simulink model "FuzzyController_SCARA"  (R2023b)
settings: Solver=VariableStepAuto  StartTime=0.0  StopTime=25  RelTol=1e-3
libraries: fuzblock x1
settings Model: Creator=Hamid Reza  LastModifiedBy=Hamid Reza

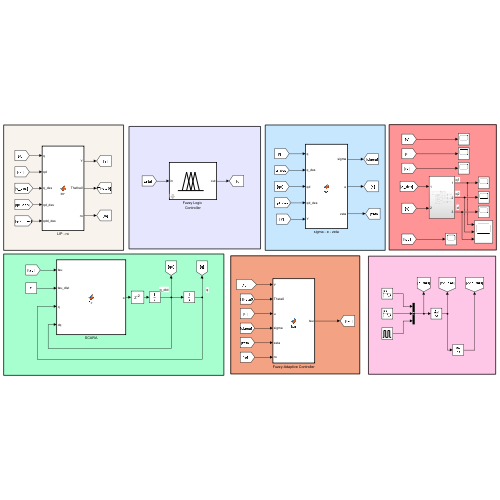
[thumbnail: Simulink's stored preview of the top-level diagram]
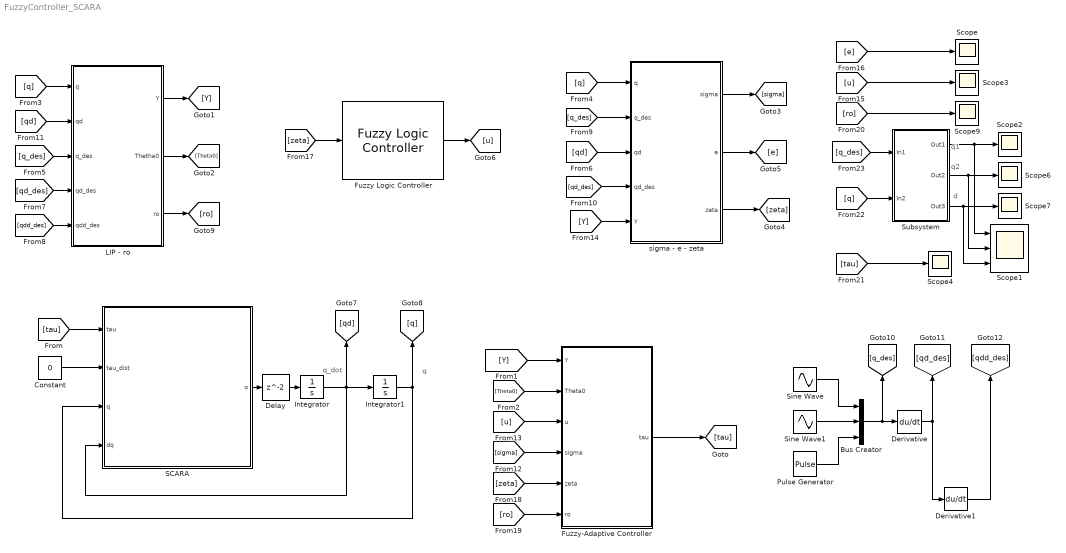
== system FuzzyController_SCARA ==
  note: q_dot
  note: q
  note: q2
  note: d
  note: q1
  Bus Creator : BusCreator  Inputs=3
  Constant : Constant  Value=0
  Delay : Delay
  Derivative : Derivative
  Derivative1 : Derivative
  Fuzzy Logic Controller : fuzblock/Fuzzy Logic  Controller  FIS='scara.fis'  OutputSampleNumber=101  DataType=double  FuzzifiedInputs=off  RuleFiringStrengths=off  RuleOutputs=off  AggregatedOutputs=off  SimulateUsing=Interpreted execution  OutOfRangeInputValueMessage=warning  NoRuleFiredMessage=warning  EmptyOutputFuzzySetMessage=warning
  Fuzzy-Adaptive Controller : MATLAB Function  TreatAsAtomicUnit=on
  Integrator : Integrator  InitialCondition=zeros(3,1)
  Integrator1 : Integrator  InitialCondition=zeros(3,1)
  LIP - ro : MATLAB Function  TreatAsAtomicUnit=on
  Pulse Generator : DiscretePulseGenerator  PulseType=Time based  Period=5  PulseWidth=50
  SCARA : MATLAB Function  TreatAsAtomicUnit=on
  Scope{,2..4,6..7,9} (7 alike) : Scope
  Scope1 : Scope  NumInputPorts=3
  Sine Wave : Sin  Frequency=5  SampleTime=0
  Sine Wave1 : Sin  Frequency=5  Phase=pi/2  SampleTime=0
  Subsystem : Subsystem
  sigma - e - zeta : MATLAB Function  TreatAsAtomicUnit=on
  wires:
  Integrator1/1 -> SCARA/3(q), [q]
  Integrator/1 -> SCARA/4(dq), Integrator1/1, [qd]
  Constant/1 -> SCARA/2(tau_dist)
  [tau] -> SCARA/1(tau)
  Fuzzy-Adaptive Controller/1(tau) -> [tau]
  [Y] -> Fuzzy-Adaptive Controller/1(Y)
  [Theta0] -> Fuzzy-Adaptive Controller/2(Theta0)
  [q] -> sigma - e - zeta/1(q)
  [qd] -> sigma - e - zeta/3(qd)
  [q_des] -> sigma - e - zeta/2(q_des)
  sigma - e - zeta/1(sigma) -> [sigma]
  sigma - e - zeta/2(e) -> [e]
  [qd_des] -> sigma - e - zeta/4(qd_des)
  Sine Wave/1 -> Bus Creator/1
  Sine Wave1/1 -> Bus Creator/2
  Bus Creator/1 -> [q_des], Derivative/1
  Derivative/1 -> Derivative1/1, [qd_des]
  Derivative1/1 -> [qdd_des]
  Pulse Generator/1 -> Bus Creator/3
  [e] -> Scope/1
  [tau] -> Scope4/1
  [q_des] -> Subsystem/1(In1)
  [q] -> Subsystem/2(In2)
  Subsystem/1(Out1) -> Scope2/1, Scope1/1
  Subsystem/2(Out2) -> Scope1/2, Scope6/1
  Subsystem/3(Out3) -> Scope1/3, Scope7/1
  [q] -> LIP - ro/1(q)
  [qdd_des] -> LIP - ro/5(qdd_des)
  [qd_des] -> LIP - ro/4(qd_des)
  [q_des] -> LIP - ro/3(q_des)
  [qd] -> LIP - ro/2(qd)
  LIP - ro/2(Thetha0) -> [Theta0]
  LIP - ro/1(Y) -> [Y]
  [sigma] -> Fuzzy-Adaptive Controller/4(sigma)
  [u] -> Fuzzy-Adaptive Controller/3(u)
  [Y] -> sigma - e - zeta/5(Y)
  sigma - e - zeta/3(zeta) -> [zeta]
  Fuzzy Logic Controller/1 -> [u]
  [zeta] -> Fuzzy Logic Controller/1
  [u] -> Scope3/1
  [zeta] -> Fuzzy-Adaptive Controller/5(zeta)
  SCARA/1(o) -> Delay/1
  Delay/1 -> Integrator/1
  [ro] -> Fuzzy-Adaptive Controller/6(ro)
  LIP - ro/3(ro) -> [ro]
  [ro] -> Scope9/1

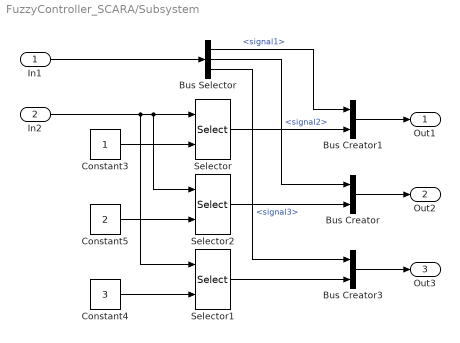
== system FuzzyController_SCARA/Subsystem ==
  In1 : Inport
  In2 : Inport  Port=2
  Bus Creator : BusCreator  Inputs=2
  Bus Creator1 : BusCreator  Inputs=2
  Bus Creator3 : BusCreator  Inputs=2
  Bus Selector : BusSelector  OutputSignals=signal1,signal2,signal3
  Constant3 : Constant
  Constant4 : Constant  Value=3
  Constant5 : Constant  Value=2
  Selector : Selector  InputPortWidth=3  IndexOptions=Index vector (port)  Indices=1  OutputSizes=1
  Selector1 : Selector  InputPortWidth=3  IndexOptions=Index vector (port)  Indices=1  OutputSizes=1
  Selector2 : Selector  InputPortWidth=3  IndexOptions=Index vector (port)  Indices=1  OutputSizes=1
  Out1 : Outport
  Out2 : Outport  Port=2
  Out3 : Outport  Port=3
  wires:
  Bus Selector/3 -> Bus Creator3/1  "<signal3>"
  Bus Selector/2 -> Bus Creator/1  "<signal2>"
  Selector2/1 -> Bus Creator/2
  Constant3/1 -> Selector/2
  Selector/1 -> Bus Creator1/2
  Bus Selector/1 -> Bus Creator1/1  "<signal1>"
  Bus Creator3/1 -> Out3/1
  Selector1/1 -> Bus Creator3/2
  Constant5/1 -> Selector2/2
  Constant4/1 -> Selector1/2
  In2/1 -> Selector1/1, Selector2/1, Selector/1
  Bus Creator/1 -> Out2/1
  Bus Creator1/1 -> Out1/1
  In1/1 -> Bus Selector/1

== matlab function FuzzyController_SCARA/Fuzzy-Adaptive Controller ==
  data: Y input; tau output; Theta0 input; u input; sigma input; zeta input; ro input
function tau = fcn(Y, Theta0, u, sigma, zeta, ro)

tau = (Y*(Theta0 - u)) - K_adaptive(sigma,[0.000001;0.000001;0.000001],zeta,u, ro)*sigma ;



function K = K_adaptive (sigma, epsilon, zeta, u, ro)

    if sigma > epsilon
       K1 = max((abs(zeta).*abs(ro-u))/sigma(1)^2)  ;
       K2 = max((abs(zeta).*abs(ro-u))/sigma(2)^2)  ;
       K3 = max((abs(zeta).*abs(ro-u))/sigma(3)^2)  ;
       K = diag([K1, K2, K3]);
    else
       K = max( (abs(zeta).*abs(ro-u))/epsilon) ;
       K = diag(K);
    end
end

end

== matlab function FuzzyController_SCARA/SCARA ==
  data: tau input; tau_dist input; q input; dq input; o output
function o  = fcn(tau,tau_dist,q,dq)



theta1=q(1);
theta2=q(2);
d=q(3);

dtheta1=dq(1);
dtheta2=dq(2);
dd=dq(3);


a1=0.6;
a2=0.4;
m1=12;
m2=6;
m3=6;
g = 9.81;


% define mass matrix

m11 = (1/3)*m1*a1^2+m2*(a1^2+(1/3)*a2^2+a1*a2*cos(theta2))+m3*(a1^2+a2^2+2*a1*a2*cos(theta2));
m12 = -m2*a2*((1/3)*a2+(1/2)*a1*cos(theta2))-m3*(a2^2+a1*a2*cos(theta2));
m13 = 0;
m21 = m12;
m22 = (1/3)*m2*a2^2+m3*(a2^2);
m23 = 0;
m31 = m13;
m32 = m23;
m33 = m3;

M = [m11,m12,m13;m21,m22,m23;m31,m32,m33];


% define gravity matrix

g = [0; 0; -m3*g];

% define coriolis and centrifugal matrix

c1 = -(m2+2*m3)*a1*a2*sin(theta2)*(dtheta1*dtheta2+((1/2)*dtheta2^2));
c2 = ((1/2)*m2+m3)*a1*a2*sin(theta2)*(dtheta1^2);
c3 = 0;

C = [c1 ; c2 ; c3];


o=pinv(M)*(tau+tau_dist-(C+g));

== matlab function FuzzyController_SCARA/LIP - ro ==
  data: q input; Y output; qd input; q_des input; Thetha0 output; qd_des input; qdd_des input; ro output
function [Y, Thetha0, ro] = fcn(q, qd, q_des, qd_des, qdd_des)

qd_r = qd_des - diag(4015)*(q_des-q);
qdd_r = qdd_des - diag(4015)*(qd_des-qd);

theta1=q(1);
theta2=q(2);
d=q(3);

dtheta1=qd(1);
dtheta2=qd(2);
dd=qd(3);

dtheta1_r=qd_r(1);
dtheta2_r=qd_r(2);
dd_r=qd_r(3);


ddtheta1_r=qdd_r(1);
ddtheta2_r=qdd_r(2);
ddd_r=qdd_r(3);



% Initial Values (close to Real values)
a1_0=0.5;
a2_0=0.5;
m1_0=10;
m2_0=7;
m3_0=5.5;
g = 9.81;


% Main Lagrange equations

tau1 = (((1/3)*m1_0+m2_0+m3_0)*a1_0^2+(m2_0+2*m3_0)*(a1_0*a2_0*cos(theta2))+((1/3)*m2_0+m3_0)*a2_0^2)*ddtheta1_r+((1/2)*m2_0+m3_0*a1_0*a2_0*cos(theta2)+((1/3)*m2_0+m3_0)*a2_0^2)*ddtheta2_r-(m2_0+2*m3_0)*a1_0*a2_0*sin(theta2)*(dtheta2_r*dtheta1_r+0.5*dtheta2_r^2);
tau2 = ((0.5*m2_0+m3_0)*a1_0*a2_0*cos(theta2)+((1/3)*m2_0+m3_0)*a2_0^2)*ddtheta1_r + ((1/3)*m2_0+m3_0)*a2_0^2*ddtheta2_r + (0.5*m2_0+m3_0)*a1_0*a2_0*sin(theta2)*dtheta1_r^2 ;
f = m3_0*ddd_r - m3_0*g ;


% Calculate LIP for Y and Thetha0

thetha01 = [ ((1/3)*m1_0+m2_0+m3_0)*a1_0^2 ; (m2_0+2*m3_0)*a1_0*a2_0 ; (1/3)*m2_0+m3_0*a2_0^2 ; ((1/2)*m2_0+m3_0)*a1_0*a2_0 ; ((1/3)*m2_0+m3_0)*a2_0^2 ; -(m2_0+2*m3_0)*a1_0*a2_0];
y1 = [ddtheta1_r,ddtheta1_r*cos(theta2),ddtheta1_r,ddtheta2_r*cos(theta2),ddtheta2_r,sin(theta2)*(dtheta1_r*dtheta2_r+0.5*dtheta2_r*dtheta2)];

thetha02 = [ (0.5*m2_0+m3_0)*a1_0*a2_0 ; ((1/3)*m2_0+m3_0)*a2_0^2 ; ((1/3)*m2_0+m3_0)*a2_0^2 ; (0.5*m2_0+m3_0)*a1_0*a2_0 ];
 y2 = [ddtheta1_r*cos(theta2),ddtheta1_r,ddtheta2_r,sin(theta2)*dtheta1_r*dtheta1];


thetha03  = [m3_0 ; -m3_0];
 y3 = [ddd_r , g];

Thetha0 = [thetha01;thetha02;thetha03];
Y = [y1,0,0,0,0,0,0;0,0,0,0,0,0,y2,0,0;0,0,0,0,0,0,0,0,0,0,y3];



 % Calculate Thetha and ro(Upper Uncertainly Bound)

a1=0.6;
a2=0.4;
m1=12;
m2=6;
m3=6;
g = 9.81;

thetha1 = [ ((1/3)*m1+m2+m3)*a1^2 ; (m2+2*m3)*a1*a2 ; (1/3)*m2+m3*a2^2 ; ((1/2)*m2+m3)*a1*a2 ; ((1/3)*m2+m3)*a2^2 ; -(m2+2*m3)*a1*a2];
thetha2 = [ (0.5*m2+m3)*a1*a2 ; ((1/3)*m2+m3)*a2^2 ; ((1/3)*m2+m3)*a2^2 ; (0.5*m2+m3)*a1*a2];
thetha3  = [m3 ; -m3];

Thetha = [thetha1;thetha2;thetha3];

ro = abs(Thetha - Thetha0);

== matlab function FuzzyController_SCARA/sigma - e - zeta ==
  data: q input; q_des input; sigma output; qd input; qd_des input; e output; zeta output; Y input
function [sigma,e,zeta] = fcn(q,q_des,qd,qd_des,Y)
qd_r = qd_des - 80*(q-q_des);
e = q_des - q;
sigma = qd - qd_r;
zeta = Y'*sigma;
